simulink model "chap6_2sim"  (Simulink 8.3)
settings: Solver=ode45  StartTime=0.0  StopTime=10  RelTol=1e-3
settings Model: Creator=liujk  LastModifiedBy=Prof_Liu  ExtModeTrigMode=oneshot  ExtModeArmWhenConnect=off
settings DataIOCC: LimitDataPoints=off  SignalLoggingName=sigsOut
settings OptimizationCC: BooleanDataType=off
settings DebuggingCC: SaveWithParameterizedLinksMsg=none  SignalResolutionControl=TryResolveAllWithWarning  SolverPrmCheckMsg=none  MultiTaskDSMMsg=warning  MultiTaskCondExecSysMsg=none
settings HardwareCC: TargetUnknown=on
settings RTWCC: IncludeERTFirstTime=on

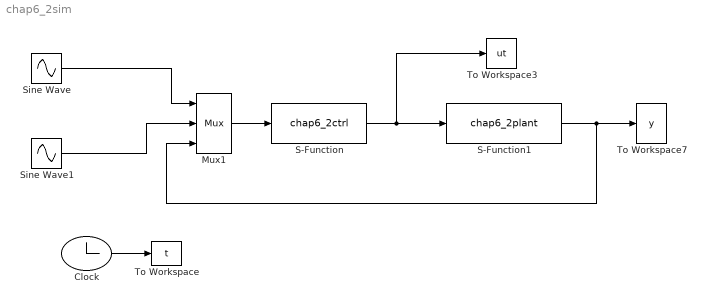
== system chap6_2sim ==
  Clock : Clock
  Mux1 : Mux  Inputs=3
  S-Function : S-Function  FunctionName=chap6_2ctrl  EnableBusSupport=off
  S-Function1 : S-Function  FunctionName=chap6_2plant  EnableBusSupport=off
  Sine Wave : Sin  Amplitude=0.3  SampleTime=0
  Sine Wave1 : Sin  Amplitude=0.3  SampleTime=0
  To Workspace : ToWorkspace  VariableName=t  SampleTime=-1
  To Workspace3 : ToWorkspace  VariableName=ut  SampleTime=-1
  To Workspace7 : ToWorkspace  VariableName=y  SampleTime=-1
  wires:
  Clock/1 -> To Workspace/1
  S-Function/1 -> S-Function1/1, To Workspace3/1
  Sine Wave/1 -> Mux1/1
  Sine Wave1/1 -> Mux1/2
  S-Function1/1 -> Mux1/3, To Workspace7/1
  Mux1/1 -> S-Function/1
